simulink model "ThdRwRtStRclCmdSrvCal"  (R2024b)
settings: Solver=FixedStepDiscrete  StartTime=0.0  StopTime=10.0  FixedStep=0.01  RelTol=1e-3
undefined symbols (not defined in the file or in its folder): KeSMSwPosInvalidVal_Val, PowerMode1
settings Model: Creator=sn2xws  LastModifiedBy=sn55gm
settings SolverCC: AlgebraicLoopSolver=TrustRegion
settings DataIOCC: SaveFormat=StructureWithTime  ReturnWorkspaceOutputs=off
settings OptimizationCC: DefaultParameterBehavior=Inlined  EnhancedBackFolding=on  PassReuseOutputArgsAs=Individual arguments  ZeroExternalMemoryAtStartup=off  ZeroInternalMemoryAtStartup=off  OptimizeBlockOrder=speed  DifferentSizesBufferReuse=on  OptimizationCustomize=off  EfficientTunableParamExpr=on
settings DebuggingCC: ParameterTunabilityLossMsg=error  UnconnectedInputMsg=warning  UnconnectedOutputMsg=warning  UnconnectedLineMsg=warning  ArithmeticOperatorsInVariantConditions=warning
settings ModelReferenceCC: EnableRefExpFcnMdlSchedulingChecks=on  ModelReferenceNumInstancesAllowed=Single
settings SFSimCC: MATLABDynamicMemAlloc=off  CustomCodeUndefinedFunction=UseInterfaceOnly
settings RTWCC: Description=AUTOSAR  SystemTargetFile=autosar.tlc  GenCodeOnly=on  TemplateMakefile=ert_default_tmf  GenerateReport=on  IncludeHyperlinkInReport=on  LaunchReport=on  DataTypeReplacement=CDataTypesFixedWidth  GenerateTraceInfo=on  GenerateTraceReport=on  GenerateTraceReportSl=on  GenerateTraceReportSf=on  GenerateTraceReportEml=on  GenerateCodeMetricsReport=on  GPUComputeCapability=3.5
settings CodeAppCC: ForceParamTrailComments=on  IgnoreCustomStorageClasses=off  OperatorAnnotations=on  SimulinkDataObjDesc=on  SFDataObjDesc=on  InsertBlockDesc=on
settings STFCustomTargetCC: TargetLangStandard=C99 (ISO)  MultiwordLength=256  ParMdlRefBuildCompliant=on  CompOptLevelCompliant=on  IncludeMdlTerminateFcn=off  CombineOutputUpdateFcns=on  SuppressErrorStatus=on  ERTCustomFileBanners=on  SupportNonFinite=off  SupportComplex=off  SupportContinuousTime=off  SupportNonInlinedSFcns=off  RemoveResetFunc=on  MATLABClassNameForMDSCustomization=Simulink.SoftwareTarget.ERTCustomization  AutosarCompliant=on  UseToolchainInfoCompliant=on  LookupTableObjectStructAxisOrder=2,1,3,4,...  LUTObjectStructOrderEvenSpacing=Size,Table,Breakpoints  SystemTargetFile=autosar.tlc
settings ERTTargetCC: TargetLangStandard=C99 (ISO)  ConcurrentExecutionCompliant=off  IncludeMdlTerminateFcn=off  SuppressErrorStatus=on  SupportNonFinite=off  SupportComplex=off  ModelStepFunctionPrototypeControlCompliant=off  CPPClassGenCompliant=off  AutosarCompliant=on  LookupTableObjectStructAxisOrder=2,1,3,4,...  LUTObjectStructOrderEvenSpacing=Size,Table,Breakpoints  ERTCustomFileTemplate=example_file_process.tlc  ERTFilePackagingFormat=Compact  BooleanTrueId=TRUE  BooleanFalseId=FALSE  DynamicArrayContainerType=coder::array

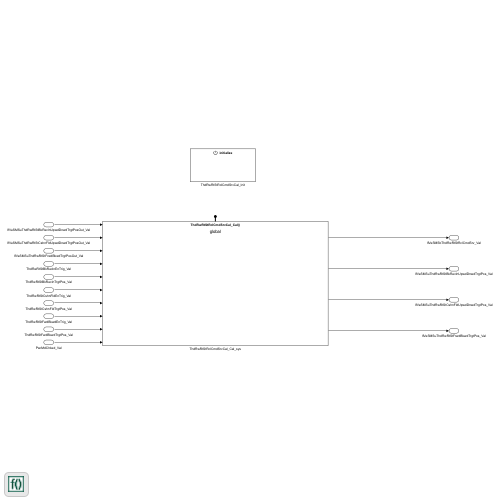
[thumbnail: Simulink's stored preview of the top-level diagram]
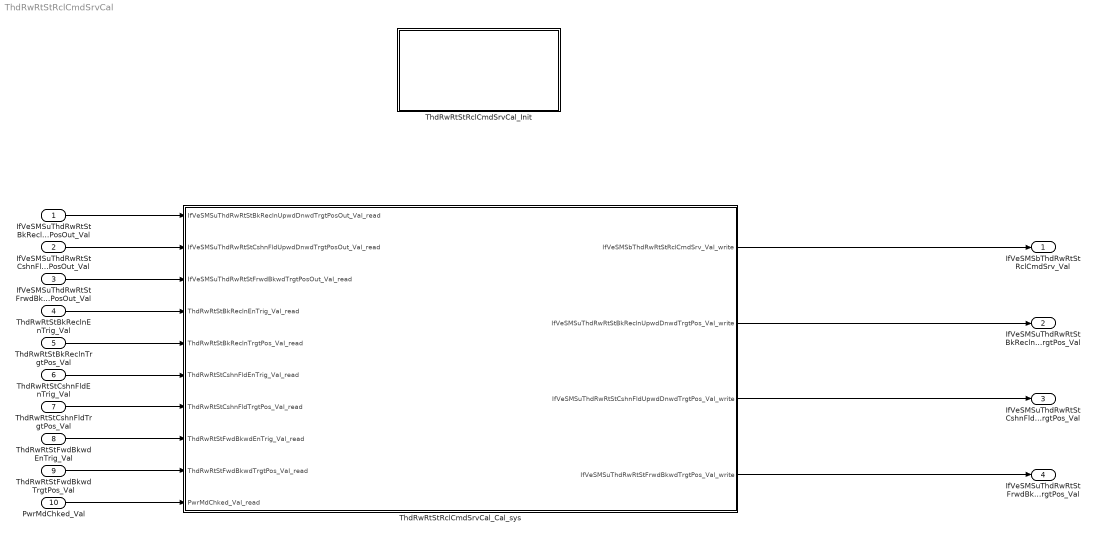
== system ThdRwRtStRclCmdSrvCal ==
  IfVeSMSuThdRwRtStBkReclnUpwdDnwdTrgtPosOut_Val : Inport  OutDataTypeStr=boolean  PortDimensions=1
  IfVeSMSuThdRwRtStCshnFldUpwdDnwdTrgtPosOut_Val : Inport  Port=2  OutDataTypeStr=boolean  PortDimensions=1
  IfVeSMSuThdRwRtStFrwdBkwdTrgtPosOut_Val : Inport  Port=3  OutDataTypeStr=boolean  PortDimensions=1
  ThdRwRtStBkReclnEnTrig_Val : Inport  Port=4  OutDataTypeStr=boolean  PortDimensions=1
  ThdRwRtStBkReclnTrgtPos_Val : Inport  Port=5  OutDataTypeStr=uint16  PortDimensions=1
  ThdRwRtStCshnFldEnTrig_Val : Inport  Port=6  OutDataTypeStr=boolean  PortDimensions=1
  ThdRwRtStCshnFldTrgtPos_Val : Inport  Port=7  OutDataTypeStr=uint16  PortDimensions=1
  ThdRwRtStFwdBkwdEnTrig_Val : Inport  Port=8  OutDataTypeStr=boolean  PortDimensions=1
  ThdRwRtStFwdBkwdTrgtPos_Val : Inport  Port=9  OutDataTypeStr=uint16  PortDimensions=1
  PwrMdChked_Val : Inport  Port=10  OutDataTypeStr=Enum: PowerMode1  PortDimensions=1
  ThdRwRtStRclCmdSrvCal_Cal_sys : Subsystem
  ThdRwRtStRclCmdSrvCal_Init : Subsystem
  IfVeSMSbThdRwRtStRclCmdSrv_Val : Outport  OutDataTypeStr=boolean  PortDimensions=1  VectorParamsAs1DForOutWhenUnconnected=off
  IfVeSMSuThdRwRtStBkReclnUpwdDnwdTrgtPos_Val : Outport  Port=2  OutDataTypeStr=uint16  PortDimensions=1  VectorParamsAs1DForOutWhenUnconnected=off
  IfVeSMSuThdRwRtStCshnFldUpwdDnwdTrgtPos_Val : Outport  Port=3  OutDataTypeStr=uint16  PortDimensions=1  VectorParamsAs1DForOutWhenUnconnected=off
  IfVeSMSuThdRwRtStFrwdBkwdTrgtPos_Val : Outport  Port=4  OutDataTypeStr=uint16  PortDimensions=1  VectorParamsAs1DForOutWhenUnconnected=off
  wires:
  IfVeSMSuThdRwRtStBkReclnUpwdDnwdTrgtPosOut_Val/1 -> ThdRwRtStRclCmdSrvCal_Cal_sys/1(IfVeSMSuThdRwRtStBkReclnUpwdDnwdTrgtPosOut_Val_read)
  IfVeSMSuThdRwRtStCshnFldUpwdDnwdTrgtPosOut_Val/1 -> ThdRwRtStRclCmdSrvCal_Cal_sys/2(IfVeSMSuThdRwRtStCshnFldUpwdDnwdTrgtPosOut_Val_read)
  IfVeSMSuThdRwRtStFrwdBkwdTrgtPosOut_Val/1 -> ThdRwRtStRclCmdSrvCal_Cal_sys/3(IfVeSMSuThdRwRtStFrwdBkwdTrgtPosOut_Val_read)
  ThdRwRtStBkReclnEnTrig_Val/1 -> ThdRwRtStRclCmdSrvCal_Cal_sys/4(ThdRwRtStBkReclnEnTrig_Val_read)
  ThdRwRtStBkReclnTrgtPos_Val/1 -> ThdRwRtStRclCmdSrvCal_Cal_sys/5(ThdRwRtStBkReclnTrgtPos_Val_read)
  ThdRwRtStCshnFldEnTrig_Val/1 -> ThdRwRtStRclCmdSrvCal_Cal_sys/6(ThdRwRtStCshnFldEnTrig_Val_read)
  ThdRwRtStCshnFldTrgtPos_Val/1 -> ThdRwRtStRclCmdSrvCal_Cal_sys/7(ThdRwRtStCshnFldTrgtPos_Val_read)
  ThdRwRtStFwdBkwdEnTrig_Val/1 -> ThdRwRtStRclCmdSrvCal_Cal_sys/8(ThdRwRtStFwdBkwdEnTrig_Val_read)
  ThdRwRtStFwdBkwdTrgtPos_Val/1 -> ThdRwRtStRclCmdSrvCal_Cal_sys/9(ThdRwRtStFwdBkwdTrgtPos_Val_read)
  ThdRwRtStRclCmdSrvCal_Cal_sys/1(IfVeSMSbThdRwRtStRclCmdSrv_Val_write) -> IfVeSMSbThdRwRtStRclCmdSrv_Val/1
  ThdRwRtStRclCmdSrvCal_Cal_sys/2(IfVeSMSuThdRwRtStBkReclnUpwdDnwdTrgtPos_Val_write) -> IfVeSMSuThdRwRtStBkReclnUpwdDnwdTrgtPos_Val/1
  ThdRwRtStRclCmdSrvCal_Cal_sys/3(IfVeSMSuThdRwRtStCshnFldUpwdDnwdTrgtPos_Val_write) -> IfVeSMSuThdRwRtStCshnFldUpwdDnwdTrgtPos_Val/1
  ThdRwRtStRclCmdSrvCal_Cal_sys/4(IfVeSMSuThdRwRtStFrwdBkwdTrgtPos_Val_write) -> IfVeSMSuThdRwRtStFrwdBkwdTrgtPos_Val/1
  PwrMdChked_Val/1 -> ThdRwRtStRclCmdSrvCal_Cal_sys/10(PwrMdChked_Val_read)

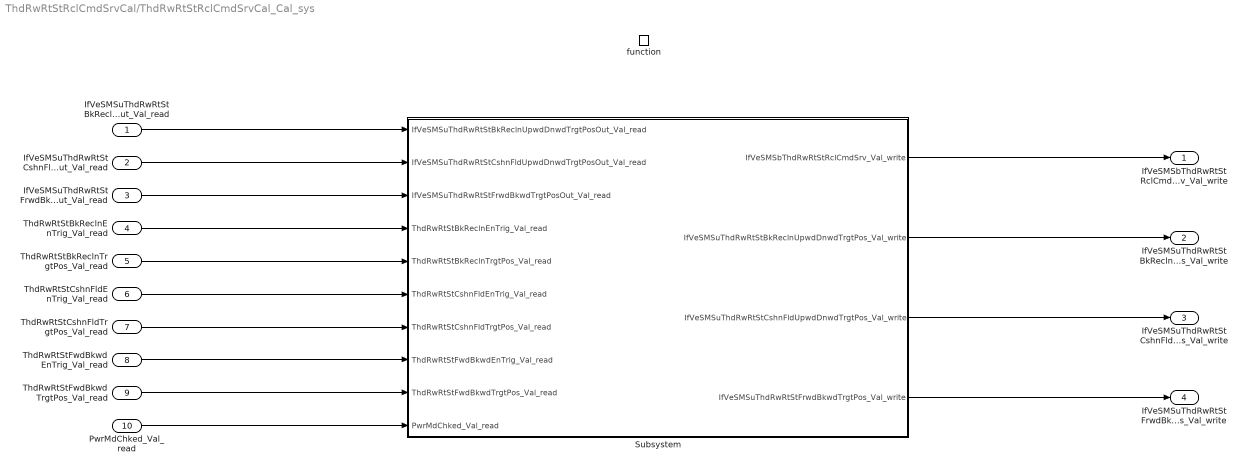
== system ThdRwRtStRclCmdSrvCal/ThdRwRtStRclCmdSrvCal_Cal_sys ==
  IfVeSMSuThdRwRtStBkReclnUpwdDnwdTrgtPosOut_Val_read : Inport
  IfVeSMSuThdRwRtStCshnFldUpwdDnwdTrgtPosOut_Val_read : Inport  Port=2
  IfVeSMSuThdRwRtStFrwdBkwdTrgtPosOut_Val_read : Inport  Port=3
  ThdRwRtStBkReclnEnTrig_Val_read : Inport  Port=4
  ThdRwRtStBkReclnTrgtPos_Val_read : Inport  Port=5
  ThdRwRtStCshnFldEnTrig_Val_read : Inport  Port=6
  ThdRwRtStCshnFldTrgtPos_Val_read : Inport  Port=7
  ThdRwRtStFwdBkwdEnTrig_Val_read : Inport  Port=8
  ThdRwRtStFwdBkwdTrgtPos_Val_read : Inport  Port=9
  PwrMdChked_Val_read : Inport  Port=10
  function : TriggerPort  TriggerType=function-call  IsSimulinkFunction=on  FunctionName=ThdRwRtStRclCmdSrvCal_Cal  VariantControl=(inherit)
  Subsystem : Subsystem
  IfVeSMSbThdRwRtStRclCmdSrv_Val_write : Outport  VectorParamsAs1DForOutWhenUnconnected=off
      settings: EnsureOutportIsVirtual=on
  IfVeSMSuThdRwRtStBkReclnUpwdDnwdTrgtPos_Val_write : Outport  Port=2  VectorParamsAs1DForOutWhenUnconnected=off
      settings: EnsureOutportIsVirtual=on
  IfVeSMSuThdRwRtStCshnFldUpwdDnwdTrgtPos_Val_write : Outport  Port=3  VectorParamsAs1DForOutWhenUnconnected=off
      settings: EnsureOutportIsVirtual=on
  IfVeSMSuThdRwRtStFrwdBkwdTrgtPos_Val_write : Outport  Port=4  VectorParamsAs1DForOutWhenUnconnected=off
      settings: EnsureOutportIsVirtual=on
  wires:
  Subsystem/1(IfVeSMSbThdRwRtStRclCmdSrv_Val_write) -> IfVeSMSbThdRwRtStRclCmdSrv_Val_write/1
  Subsystem/2(IfVeSMSuThdRwRtStBkReclnUpwdDnwdTrgtPos_Val_write) -> IfVeSMSuThdRwRtStBkReclnUpwdDnwdTrgtPos_Val_write/1
  Subsystem/3(IfVeSMSuThdRwRtStCshnFldUpwdDnwdTrgtPos_Val_write) -> IfVeSMSuThdRwRtStCshnFldUpwdDnwdTrgtPos_Val_write/1
  Subsystem/4(IfVeSMSuThdRwRtStFrwdBkwdTrgtPos_Val_write) -> IfVeSMSuThdRwRtStFrwdBkwdTrgtPos_Val_write/1
  IfVeSMSuThdRwRtStCshnFldUpwdDnwdTrgtPosOut_Val_read/1 -> Subsystem/2(IfVeSMSuThdRwRtStCshnFldUpwdDnwdTrgtPosOut_Val_read)
  IfVeSMSuThdRwRtStBkReclnUpwdDnwdTrgtPosOut_Val_read/1 -> Subsystem/1(IfVeSMSuThdRwRtStBkReclnUpwdDnwdTrgtPosOut_Val_read)
  IfVeSMSuThdRwRtStFrwdBkwdTrgtPosOut_Val_read/1 -> Subsystem/3(IfVeSMSuThdRwRtStFrwdBkwdTrgtPosOut_Val_read)
  ThdRwRtStBkReclnEnTrig_Val_read/1 -> Subsystem/4(ThdRwRtStBkReclnEnTrig_Val_read)
  ThdRwRtStBkReclnTrgtPos_Val_read/1 -> Subsystem/5(ThdRwRtStBkReclnTrgtPos_Val_read)
  ThdRwRtStCshnFldEnTrig_Val_read/1 -> Subsystem/6(ThdRwRtStCshnFldEnTrig_Val_read)
  ThdRwRtStCshnFldTrgtPos_Val_read/1 -> Subsystem/7(ThdRwRtStCshnFldTrgtPos_Val_read)
  ThdRwRtStFwdBkwdEnTrig_Val_read/1 -> Subsystem/8(ThdRwRtStFwdBkwdEnTrig_Val_read)
  ThdRwRtStFwdBkwdTrgtPos_Val_read/1 -> Subsystem/9(ThdRwRtStFwdBkwdTrgtPos_Val_read)
  PwrMdChked_Val_read/1 -> Subsystem/10(PwrMdChked_Val_read)

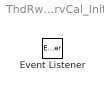
== system ThdRwRtStRclCmdSrvCal/ThdRwRtStRclCmdSrvCal_Init ==
  Event Listener : EventListener  EventName=reset

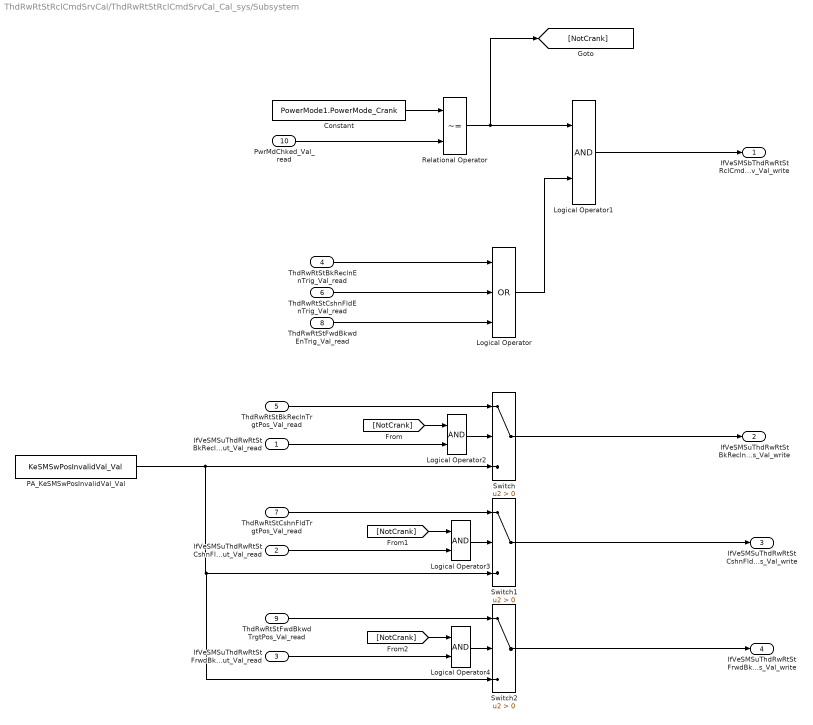
== system ThdRwRtStRclCmdSrvCal/ThdRwRtStRclCmdSrvCal_Cal_sys/Subsystem ==
  IfVeSMSuThdRwRtStBkReclnUpwdDnwdTrgtPosOut_Val_read : Inport
  IfVeSMSuThdRwRtStCshnFldUpwdDnwdTrgtPosOut_Val_read : Inport  Port=2
  IfVeSMSuThdRwRtStFrwdBkwdTrgtPosOut_Val_read : Inport  Port=3
  ThdRwRtStBkReclnEnTrig_Val_read : Inport  Port=4
  ThdRwRtStBkReclnTrgtPos_Val_read : Inport  Port=5
  ThdRwRtStCshnFldEnTrig_Val_read : Inport  Port=6
  ThdRwRtStCshnFldTrgtPos_Val_read : Inport  Port=7
  ThdRwRtStFwdBkwdEnTrig_Val_read : Inport  Port=8
  ThdRwRtStFwdBkwdTrgtPos_Val_read : Inport  Port=9
  PwrMdChked_Val_read : Inport  Port=10
  Constant : Constant  Value=PowerMode1.PowerMode_Crank  OutDataTypeStr=Enum: PowerMode1
  Logical Operator : Logic  Operator=OR  Inputs=3  AllPortsSameDT=off  OutDataTypeStr=boolean
  Logical Operator{1..4} (4 alike) : Logic  AllPortsSameDT=off  OutDataTypeStr=boolean
  PA_KeSMSwPosInvalidVal_Val : Constant  Value=KeSMSwPosInvalidVal_Val
  Relational Operator : RelationalOperator  Operator=~=  OutDataTypeStr=boolean  RndMeth=Simplest  InputSameDT=off
  Switch : Switch  Criteria=u2 > Threshold  SaturateOnIntegerOverflow=off  InputSameDT=off
  Switch1 : Switch  Criteria=u2 > Threshold  SaturateOnIntegerOverflow=off  InputSameDT=off
  Switch2 : Switch  Criteria=u2 > Threshold  SaturateOnIntegerOverflow=off  InputSameDT=off
  IfVeSMSbThdRwRtStRclCmdSrv_Val_write : Outport  VectorParamsAs1DForOutWhenUnconnected=off
      settings: EnsureOutportIsVirtual=on
  IfVeSMSuThdRwRtStBkReclnUpwdDnwdTrgtPos_Val_write : Outport  Port=2  VectorParamsAs1DForOutWhenUnconnected=off
      settings: EnsureOutportIsVirtual=on
  IfVeSMSuThdRwRtStCshnFldUpwdDnwdTrgtPos_Val_write : Outport  Port=3  VectorParamsAs1DForOutWhenUnconnected=off
      settings: EnsureOutportIsVirtual=on
  IfVeSMSuThdRwRtStFrwdBkwdTrgtPos_Val_write : Outport  Port=4  VectorParamsAs1DForOutWhenUnconnected=off
      settings: EnsureOutportIsVirtual=on
  wires:
  PA_KeSMSwPosInvalidVal_Val/1 -> Switch2/3, Switch1/3, Switch/3
  ThdRwRtStCshnFldTrgtPos_Val_read/1 -> Switch1/1
  Switch/1 -> IfVeSMSuThdRwRtStBkReclnUpwdDnwdTrgtPos_Val_write/1
  ThdRwRtStBkReclnEnTrig_Val_read/1 -> Logical Operator/1
  ThdRwRtStFwdBkwdEnTrig_Val_read/1 -> Logical Operator/3
  ThdRwRtStBkReclnTrgtPos_Val_read/1 -> Switch/1
  ThdRwRtStCshnFldEnTrig_Val_read/1 -> Logical Operator/2
  Switch1/1 -> IfVeSMSuThdRwRtStCshnFldUpwdDnwdTrgtPos_Val_write/1
  ThdRwRtStFwdBkwdTrgtPos_Val_read/1 -> Switch2/1
  Switch2/1 -> IfVeSMSuThdRwRtStFrwdBkwdTrgtPos_Val_write/1
  Relational Operator/1 -> [NotCrank], Logical Operator1/1
  Logical Operator1/1 -> IfVeSMSbThdRwRtStRclCmdSrv_Val_write/1
  Logical Operator/1 -> Logical Operator1/2
  Constant/1 -> Relational Operator/1
  PwrMdChked_Val_read/1 -> Relational Operator/2
  Logical Operator2/1 -> Switch/2
  IfVeSMSuThdRwRtStBkReclnUpwdDnwdTrgtPosOut_Val_read/1 -> Logical Operator2/2
  [NotCrank] -> Logical Operator2/1
  [NotCrank] -> Logical Operator3/1
  IfVeSMSuThdRwRtStCshnFldUpwdDnwdTrgtPosOut_Val_read/1 -> Logical Operator3/2
  Logical Operator3/1 -> Switch1/2
  Logical Operator4/1 -> Switch2/2
  IfVeSMSuThdRwRtStFrwdBkwdTrgtPosOut_Val_read/1 -> Logical Operator4/2
  [NotCrank] -> Logical Operator4/1
